simulink model "wheel_and_bar11"  (R2018a)
settings: Solver=VariableStepAuto  StartTime=0.0  StopTime=30  RelTol=1e-3
values from neighbouring files (symbols this model uses):
  A = [0 1 0 0 ... (first row only)    [PowerEnergyCons.m]    (also in main.m)
  B = [0 ... (first row only)    [PowerEnergyCons.m]    (also in main.m)
  betta = 1    [main.m]
  C = [1 0 0 0 ... (first row only)    [PowerEnergyCons.m]    (also in main.m)
  D = [0 ... (first row only)    [PowerEnergyCons.m]    (also in main.m)
  den_thetactrl_tf1 = [1 200 10000]    [PowerEnergyCons.m]    (also in main.m)
  den_thetactrl_tf2 = [1 -3]    [PowerEnergyCons.m]    (also in main.m)
  den_xctrl_tf = L    [PowerEnergyCons.m]    (also in main.m)
  Fmed = 0.25*User_Weight*g    (= -171.608675)    [PowerEnergyCons.m]    (also in main.m)
  Fvar = 0.1*User_Weight*g    (= -68.64347)    [PowerEnergyCons.m]    (also in main.m)
  num_thetactrl_tf1 = [1 20 101]    [PowerEnergyCons.m]    (also in main.m)
  num_thetactrl_tf2 = 60*[9.375 -3.2225]    [PowerEnergyCons.m]    (also in main.m)
  num_xctrl_tf = P    [PowerEnergyCons.m]    (also in main.m)
  Walking_Freq = 4    [main.m]
  X_Force = 3/sqrt(2)*sqrt(Walking_Freq)    [PowerEnergyCons.m]    (also in main.m = 4.2426)
libraries: simulink x2
settings Model: Creator=joaos  LastModifiedBy=gonca

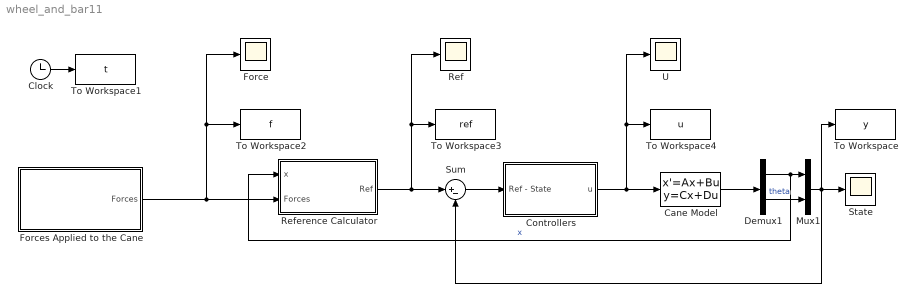
== system wheel_and_bar11 ==
  Cane Model : StateSpace  A=A  B=B  C=C  D=D  InitialCondition=0
  Clock : Clock
  Controllers : Subsystem
  Demux1 : Demux  Outputs=2
  Force : Scope
  Forces Applied to the Cane : Subsystem
  Mux1 : Mux  Inputs=2
  Ref : Scope
  Reference Calculator : Subsystem
  State : Scope
  Sum : Sum  Inputs=|+-
  To Workspace : ToWorkspace  VariableName=y  SampleTime=-1
  To Workspace1 : ToWorkspace  VariableName=t  SampleTime=-1
  To Workspace2 : ToWorkspace  VariableName=f  SampleTime=-1
  To Workspace3 : ToWorkspace  VariableName=ref  SampleTime=-1
  To Workspace4 : ToWorkspace  VariableName=u  SampleTime=-1
  U : Scope
  wires:
  Demux1/2 -> Mux1/2  "theta"
  Demux1/1 -> Reference Calculator/1(x), Mux1/1  "x"
  Cane Model/1 -> Demux1/1
  Mux1/1 -> To Workspace/1, Sum/2, State/1
  Clock/1 -> To Workspace1/1
  Forces Applied to the Cane/1(Forces) -> To Workspace2/1, Force/1, Reference Calculator/2(Forces)
  Controllers/1(u) -> Cane Model/1, U/1, To Workspace4/1
  Sum/1 -> Controllers/1(Ref - State)
  Reference Calculator/1(Ref) -> Ref/1, To Workspace3/1, Sum/1

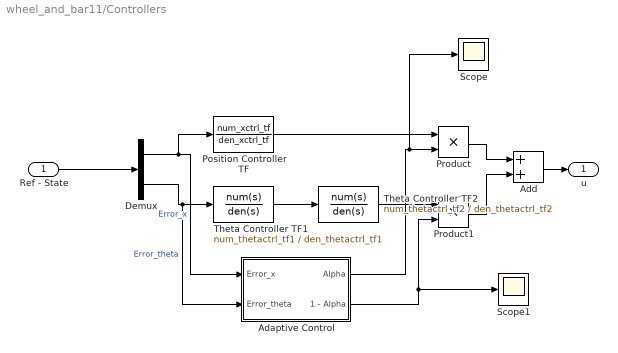
== system wheel_and_bar11/Controllers ==
  Ref - State : Inport
  Adaptive Control : Subsystem
  Add : Sum
  Demux : Demux  Outputs=2
  Position Controller TF : TransferFcn  Numerator=num_xctrl_tf  Denominator=den_xctrl_tf
  Product : Product
  Product1 : Product
  Scope : Scope
  Scope1 : Scope
  Theta Controller TF1 : TransferFcn  Numerator=num_thetactrl_tf1  Denominator=den_thetactrl_tf1
  Theta Controller TF2 : TransferFcn  Numerator=num_thetactrl_tf2  Denominator=den_thetactrl_tf2
  u : Outport
  wires:
  Theta Controller TF2/1 -> Product1/1
  Demux/1 -> Adaptive Control/1(Error_x), Position Controller TF/1  "Error_x"
  Product1/1 -> Add/2
  Demux/2 -> Adaptive Control/2(Error_theta), Theta Controller TF1/1  "Error_theta"
  Position Controller TF/1 -> Product/1
  Add/1 -> u/1
  Ref - State/1 -> Demux/1
  Theta Controller TF1/1 -> Theta Controller TF2/1
  Product/1 -> Add/1
  Adaptive Control/1(Alpha) -> Scope/1, Product/2
  Adaptive Control/2(1 - Alpha) -> Scope1/1, Product1/2

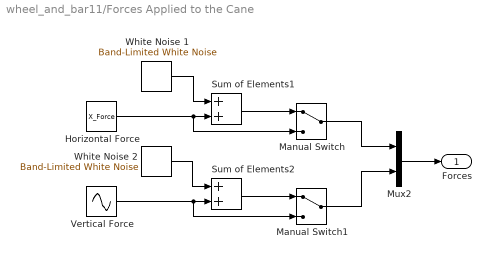
== system wheel_and_bar11/Forces Applied to the Cane ==
  Horizontal Force : Constant  Value=X_Force
  Manual Switch : ManualSwitch
  Manual Switch1 : ManualSwitch
  Mux2 : Mux  Inputs=2
  Sum of Elements1 : Sum
  Sum of Elements2 : Sum
  Vertical Force : Sin  Amplitude=Fvar  Bias=Fmed  Frequency=Walking_Freq  SampleTime=0
  White Noise 1 : simulink/Sources/Band-Limited White Noise  Cov=0.1*X_Force  Ts=0.1  seed=[23341]
  White Noise 2 : simulink/Sources/Band-Limited White Noise  Cov=-0.1*Fvar  Ts=0.1  seed=[23341]
  Forces : Outport
  wires:
  Vertical Force/1 -> Manual Switch1/2, Sum of Elements2/2
  Horizontal Force/1 -> Manual Switch/2, Sum of Elements1/2
  White Noise 2/1 -> Sum of Elements2/1
  Mux2/1 -> Forces/1
  White Noise 1/1 -> Sum of Elements1/1
  Manual Switch/1 -> Mux2/1
  Manual Switch1/1 -> Mux2/2
  Sum of Elements1/1 -> Manual Switch/1
  Sum of Elements2/1 -> Manual Switch1/1

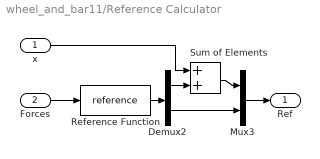
== system wheel_and_bar11/Reference Calculator ==
  x : Inport
  Forces : Inport  Port=2
  Demux2 : Demux  Outputs=2
  Mux3 : Mux  Inputs=2
  Reference Function : MATLABFcn  MATLABFcn=reference  OutputDimensions=2
  Sum of Elements : Sum
  Ref : Outport
  wires:
  Reference Function/1 -> Demux2/1
  Forces/1 -> Reference Function/1
  x/1 -> Sum of Elements/1
  Mux3/1 -> Ref/1
  Sum of Elements/1 -> Mux3/1
  Demux2/2 -> Mux3/2
  Demux2/1 -> Sum of Elements/2

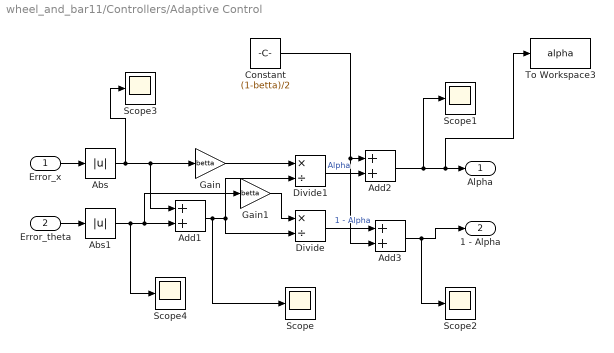
== system wheel_and_bar11/Controllers/Adaptive Control ==
  Error_x : Inport
  Error_theta : Inport  Port=2
  Abs : Abs
  Abs1 : Abs
  Add1 : Sum
  Add2 : Sum
  Add3 : Sum
  Constant : Constant  Value=(1-betta)/2
  Divide : Product  Inputs=*/
  Divide1 : Product  Inputs=*/
  Gain : Gain  Gain=betta
  Gain1 : Gain  Gain=betta
  Scope{,1..4} (5 alike) : Scope
  To Workspace3 : ToWorkspace  VariableName=alpha  SampleTime=-1
  Alpha : Outport
  1 - Alpha : Outport  Port=2
  wires:
  Error_theta/1 -> Abs1/1
  Add1/1 -> Scope/1, Divide1/2, Divide/2
  Error_x/1 -> Abs/1
  Abs/1 -> Scope3/1, Add1/1, Gain/1
  Abs1/1 -> Scope4/1, Gain1/1, Add1/2
  Gain/1 -> Divide1/1
  Gain1/1 -> Divide/1
  Add2/1 -> To Workspace3/1, Alpha/1, Scope1/1
  Divide1/1 -> Add2/2  "Alpha"
  Constant/1 -> Add3/2, Add2/1
  Divide/1 -> Add3/1  "1 - Alpha"
  Add3/1 -> Scope2/1, 1 - Alpha/1
